simulink model "new_composition"  (R2024a)
settings: Solver=FixedStepDiscrete  StartTime=0.0  StopTime=10.0  RelTol=1e-3  EnableMultiTasking=on
undefined symbols (not defined in the file or in its folder): D1, P
settings Model: DataDictionary=interfaces.sldd  Creator=Mhamed  LastModifiedBy=Mhamed
settings SolverCC: AlgebraicLoopSolver=TrustRegion  AutoInsertRateTranBlk=on  InsertRTBMode=Never (minimum delay)  MaxZcPerStep=1
settings OptimizationCC: DefaultParameterBehavior=Inlined  EnhancedBackFolding=on  PassReuseOutputArgsAs=Individual arguments  ZeroExternalMemoryAtStartup=off  ZeroInternalMemoryAtStartup=off  OptimizeBlockOrder=speed  DifferentSizesBufferReuse=on  OptimizationCustomize=off  EfficientTunableParamExpr=on
settings DebuggingCC: MultiTaskDSMMsg=none  MultiTaskRateTransMsg=warning  ParameterTunabilityLossMsg=error  UnconnectedLineMsg=warning
settings ModelReferenceCC: EnableRefExpFcnMdlSchedulingChecks=on
settings SFSimCC: MATLABDynamicMemAlloc=off
settings RTWCC: Description=AUTOSAR  SystemTargetFile=autosar.tlc  GenCodeOnly=on  TemplateMakefile=ert_default_tmf  IncludeHyperlinkInReport=on  DataTypeReplacement=CDataTypesFixedWidth  GPUComputeCapability=3.5  DLArmComputeVersion=19.05
settings CodeAppCC: ForceParamTrailComments=on  IgnoreCustomStorageClasses=off  OperatorAnnotations=on  SimulinkDataObjDesc=on  SFDataObjDesc=on  InsertBlockDesc=on
settings STFCustomTargetCC: MultiwordLength=256  ParMdlRefBuildCompliant=on  CompOptLevelCompliant=on  IncludeMdlTerminateFcn=off  CombineOutputUpdateFcns=on  SuppressErrorStatus=on  ERTCustomFileBanners=on  SupportNonFinite=off  SupportComplex=off  SupportContinuousTime=off  SupportNonInlinedSFcns=off  RemoveResetFunc=on  MATLABClassNameForMDSCustomization=Simulink.SoftwareTarget.ERTCustomization  AutosarCompliant=on  GRTInterface=off  LookupTableObjectStructAxisOrder=2,1,3,4,...  LUTObjectStructOrderEvenSpacing=Size,Table,Breakpoints  SystemTargetFile=autosar.tlc
settings ERTTargetCC: TargetLangStandard=C99 (ISO)  ConcurrentExecutionCompliant=off  IncludeMdlTerminateFcn=off  SuppressErrorStatus=on  SupportNonFinite=off  SupportComplex=off  ModelStepFunctionPrototypeControlCompliant=off  CPPClassGenCompliant=off  AutosarCompliant=on  LookupTableObjectStructAxisOrder=2,1,3,4,...  LUTObjectStructOrderEvenSpacing=Size,Table,Breakpoints  InlinedParameterPlacement=NonHierarchical  ERTCustomFileTemplate=example_file_process.tlc  BooleanTrueId=TRUE  BooleanFalseId=FALSE

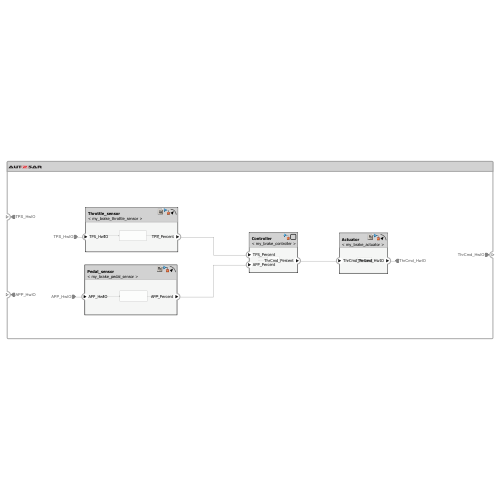
[thumbnail: Simulink's stored preview of the top-level diagram]
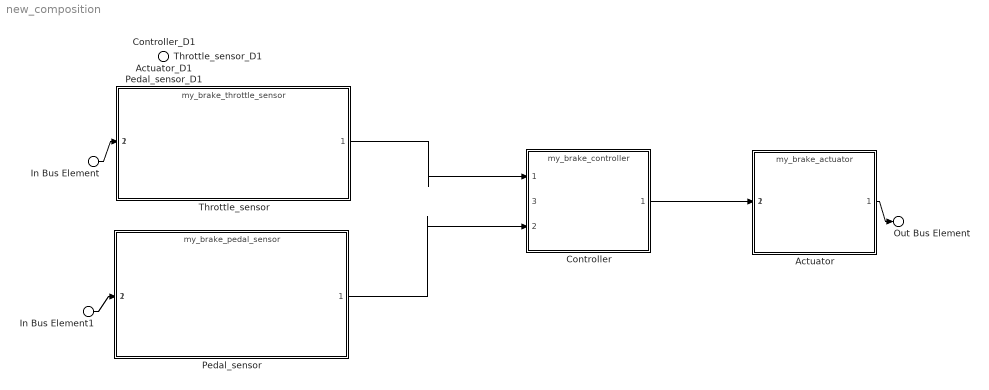
== system new_composition ==
  In Bus Element : Inport  PortName=TPS_HwIO
  In Bus Element1 : Inport  Port=2  PortName=APP_HwIO
  Actuator_D1 : Inport  Port=3  OutputFunctionCall=on
  Controller_D1 : Inport  Port=4  OutputFunctionCall=on
  Pedal_sensor_D1 : Inport  Port=5  OutputFunctionCall=on
  Throttle_sensor_D1 : Inport  Port=6  SampleTime=0.005  OutputFunctionCall=on
  Actuator : ModelReference  ModelNameDialog=my_brake_actuator  SimulationMode=Normal  ScheduleRates=on  CachedPortDiscreteRates=[0.005]  ModelEventPortInfo=P:D1[0.005][0][0]  CodeInterface=Top model  ModelReferenceVersion=9.4
      settings: PortSchema="{\"entries\":[{\"content\":{\"headerSize\":38,\"margin\":15,\"minimumSpacing\":25,\"sides\":[{\"content\":{\"connectorIds\":[\"In1\"]},\"type\":\"ConnectorPlacement.EquallySpacedRectSide\",\"uuid\":\"d23841e5-5eda-4da2-9b65-3d12d8e26663\"},{\"content\":{\"connectorIds\":[\"Out1\"],\"side\":\"RIGHT\"},\"type\":\"ConnectorPlacement.EquallySpacedRectSide\",\"uuid\":\"ce57982c-7e95-4c97-86dc-2987ef89b288\"},{\"content\":{\"side\":\"TOP\"},\"type\":\"ConnectorPlacement.EquallySpacedRectSide\",\"uuid\":\"a00580a5-5d7b-48c6-a204-81d3b2555c5f\"},{\"content\":{\"connectorIds\":[\"In2\"],\"side\":\"HIDDEN\"},\"type\":\"ConnectorPlacement.EquallySpacedRectSide\",\"uuid\":\"5ce3603b-1dd9-4dc8-a257-2a9f696276fb\"}]},\"type\":\"ConnectorPlacement.EquallySpacedConnector\",\"uuid\":\"7e8e924e-0cb8-42b6-8ff8-f4da4b4bc3d8\"}],\"packageUris\":[\"http://schema.mathworks.com/mf0/Connector/R2020b\"],\"version\":\"1.0\"}"
  Controller : ModelReference  ModelNameDialog=my_brake_controller  SimulationMode=Normal  ScheduleRates=on  CachedPortDiscreteRates=[0.005]  ModelEventPortInfo=P:D1[0.005][0][0]  CodeInterface=Top model  ModelReferenceVersion=10.4
      settings: PortSchema="{\"entries\":[{\"content\":{\"headerSize\":38,\"margin\":15,\"minimumSpacing\":25,\"sides\":[{\"content\":{\"connectorIds\":[\"In1\",\"In2\"]},\"type\":\"ConnectorPlacement.EquallySpacedRectSide\",\"uuid\":\"d23841e5-5eda-4da2-9b65-3d12d8e26663\"},{\"content\":{\"connectorIds\":[\"Out1\"],\"side\":\"RIGHT\"},\"type\":\"ConnectorPlacement.EquallySpacedRectSide\",\"uuid\":\"ce57982c-7e95-4c97-86dc-2987ef89b288\"},{\"content\":{\"side\":\"TOP\"},\"type\":\"ConnectorPlacement.EquallySpacedRectSide\",\"uuid\":\"a00580a5-5d7b-48c6-a204-81d3b2555c5f\"},{\"content\":{\"connectorIds\":[\"In3\"],\"side\":\"HIDDEN\"},\"type\":\"ConnectorPlacement.EquallySpacedRectSide\",\"uuid\":\"6c36d114-0a7b-4fac-ac8a-0f2efd6f257b\"}]},\"type\":\"ConnectorPlacement.EquallySpacedConnector\",\"uuid\":\"7e8e924e-0cb8-42b6-8ff8-f4da4b4bc3d8\"}],\"packageUris\":[\"http://schema.mathworks.com/mf0/Connector/R2020b\"],\"version\":\"1.0\"}"
  Pedal_sensor : ModelReference  ModelNameDialog=my_brake_pedal_sensor  SimulationMode=Normal  ScheduleRates=on  CachedPortDiscreteRates=[0.005]  ModelEventPortInfo=P:D1[0.005][0][0]  CodeInterface=Top model  ModelReferenceVersion=9.5
      settings: PortSchema="{\"entries\":[{\"content\":{\"headerSize\":38,\"margin\":15,\"minimumSpacing\":25,\"sides\":[{\"content\":{\"connectorIds\":[\"In1\"]},\"type\":\"ConnectorPlacement.EquallySpacedRectSide\",\"uuid\":\"d23841e5-5eda-4da2-9b65-3d12d8e26663\"},{\"content\":{\"connectorIds\":[\"Out1\"],\"side\":\"RIGHT\"},\"type\":\"ConnectorPlacement.EquallySpacedRectSide\",\"uuid\":\"ce57982c-7e95-4c97-86dc-2987ef89b288\"},{\"content\":{\"side\":\"TOP\"},\"type\":\"ConnectorPlacement.EquallySpacedRectSide\",\"uuid\":\"a00580a5-5d7b-48c6-a204-81d3b2555c5f\"},{\"content\":{\"connectorIds\":[\"In2\"],\"side\":\"HIDDEN\"},\"type\":\"ConnectorPlacement.EquallySpacedRectSide\",\"uuid\":\"c24bdfd9-e664-4be8-9fe3-6ab0a191d1a9\"}]},\"type\":\"ConnectorPlacement.EquallySpacedConnector\",\"uuid\":\"7e8e924e-0cb8-42b6-8ff8-f4da4b4bc3d8\"}],\"packageUris\":[\"http://schema.mathworks.com/mf0/Connector/R2020b\"],\"version\":\"1.0\"}"
  Throttle_sensor : ModelReference  ModelNameDialog=my_brake_throttle_sensor  UsingDefaultArgumentValue=0  SimulationMode=Normal  ScheduleRates=on  CachedPortDiscreteRates=[0.005]  ModelEventPortInfo=P:D1[0.005][0][0]  CodeInterface=Top model  ModelReferenceVersion=9.5
      settings: PortSchema="{\"entries\":[{\"content\":{\"headerSize\":38,\"margin\":15,\"minimumSpacing\":25,\"sides\":[{\"content\":{\"connectorIds\":[\"In1\"]},\"type\":\"ConnectorPlacement.EquallySpacedRectSide\",\"uuid\":\"d23841e5-5eda-4da2-9b65-3d12d8e26663\"},{\"content\":{\"connectorIds\":[\"Out1\"],\"side\":\"RIGHT\"},\"type\":\"ConnectorPlacement.EquallySpacedRectSide\",\"uuid\":\"ce57982c-7e95-4c97-86dc-2987ef89b288\"},{\"content\":{\"side\":\"TOP\"},\"type\":\"ConnectorPlacement.EquallySpacedRectSide\",\"uuid\":\"a00580a5-5d7b-48c6-a204-81d3b2555c5f\"},{\"content\":{\"connectorIds\":[\"In2\"],\"side\":\"HIDDEN\"},\"type\":\"ConnectorPlacement.EquallySpacedRectSide\",\"uuid\":\"5b982779-f5ba-43d7-aec8-fa7796851617\"}]},\"type\":\"ConnectorPlacement.EquallySpacedConnector\",\"uuid\":\"7e8e924e-0cb8-42b6-8ff8-f4da4b4bc3d8\"}],\"packageUris\":[\"http://schema.mathworks.com/mf0/Connector/R2020b\"],\"version\":\"1.0\"}"
  Out Bus Element : Outport  PortName=ThrCmd_HwIO
  wires:
  Pedal_sensor/1 -> Controller/2
  Controller/1 -> Actuator/1
  Actuator/1 -> Out Bus Element/1
  In Bus Element1/1 -> Pedal_sensor/1
  In Bus Element/1 -> Throttle_sensor/1
  Throttle_sensor/1 -> Controller/1
